simulink model "main_model"  (R2023b)
settings: Solver=FixedStepAuto  StartTime=0.0  StopTime=stopTime  RelTol=1e-3
values from neighbouring files (symbols this model uses):
  a = 6939    [Air_Drag_script.m]    (also in main.m = 6939.063; main_group24.m = 6978)
  A_BN0 = eye(3)    [main.m]
  c = 2.99792*10^8    (= 299792000)    [main.m]    (also in main_group24.m = 299792458)
  e = 0    [Air_Drag_script.m]    (also in main.m = 0.001304; main_group24.m)
  G = [gn, gm, gvali, gsvi]    [main.m]    (also in main_group24.m)
  H = [hn, hm, hvali, hsvi]    [main.m]    (also in main_group24.m)
  i = deg2rad(97.5307)    [Air_Drag_script.m]    (also in main.m; main_group24.m = deg2rad(98))
  inertia1 = Iz-Iy    (= -0.016811111)    [main.m]
  inertia2 = Ix-Iz    (= 0.033125546)    [main.m]
  inertia3 = Iy-Ix    (= -0.016314435)    [main.m]
  Inertia_matrix = [Ix 0 0; 0 Iy 0; 0 0 Iz]    [main.m]
  Inverse_inertia = inv(Inertia_matrix)    [main.m]
  m = [0.1; 0.1; 0.1]    [main.m]    (also in main_group24.m)
  MB = [4; 0.1; 0.1; 0.3]    [main.m]    (also in main_group24.m)
  mu = 3.98600433e+5    (= 398600.433)    [main.m]    (also in main_group24.m)
  n = 0.0011    [Air_Drag_script.m]    (also in main.m = sqrt(mu/a^3); main_group24.m = sqrt(mu/a^3))
  R_e = 6378    [main.m]    (also in main_group24.m)
  rho_d_MB = 0.1    [main.m]
  rho_d_SP = 0.1    [main.m]
  rho_s_MB = 0.5    [main.m]
  rho_s_SP = 0.1    [main.m]
  SP = [1; 0.3; 0.1; 0.01]    [main.m]    (also in main_group24.m = [0.25; 0.1; 0.3; 0.01])
  theta0 = deg2rad(30)    [main.m]    (also in main_group24.m = deg2rad(0))
  wx0 = deg2rad(3)    [main.m]    (also in main_group24.m)
  wy0 = deg2rad(11)    [main.m]    (also in main_group24.m)
  wz0 = deg2rad(14)    [main.m]    (also in main_group24.m)
libraries: matrix_library x8, vrlib x3, simulink_extras x1
(part 1 of 3)
settings Model: Creator=adity  LastModifiedBy=adity

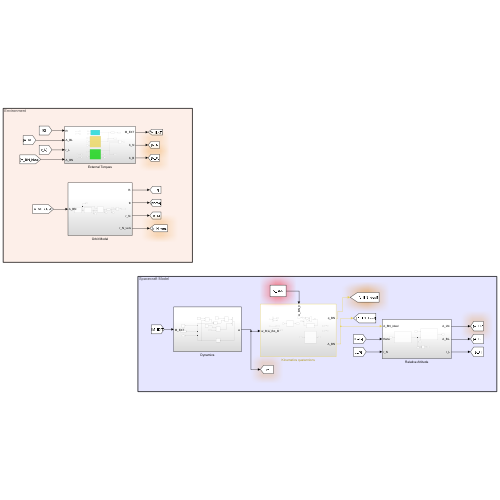
[thumbnail: Simulink's stored preview of the top-level diagram]
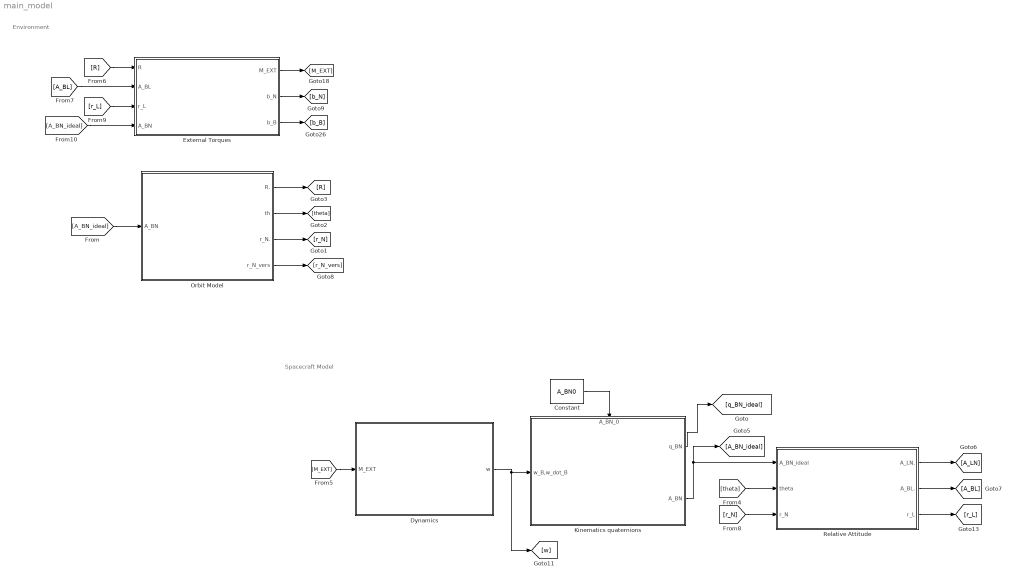
== system main_model ==
  note: Environment
  note: Spacecraft Model
  Constant : Constant  Value=A_BN0
  Dynamics : Subsystem
  External Torques : Subsystem
  Kinematics quaternions : Subsystem
      settings: PortSchema="{\"entries\":[{\"content\":{\"sides\":[{\"content\":{\"connectorIds\":[\"In1\"]},\"type\":\"ConnectorPlacement.EquallySpacedRectSide\",\"uuid\":\"b4580536-f47d-4a76-9d7a-ad9e45e6fd22\"},{\"content\":{\"connectorIds\":[\"Out1\",\"Out2\"],\"side\":\"RIGHT\"},\"type\":\"ConnectorPlacement.EquallySpacedRectSide\",\"uuid\":\"4273ed6e-d469-4a82-9e71-da4fb1c9f709\"},{\"content\":{\"connectorIds\":[\"In2\"],\"side\":\"TOP\"},\"type\":\"ConnectorPlacement.EquallySpacedRectSide\",\"uuid\":\"bac57a2b-a638-4d55-8f6f-550bb52319aa\"}]},\"type\":\"ConnectorPlacement.EquallySpacedConnector\",\"uuid\":\"29527554-7b77-4957-9d93-347c44cffae5\"}],\"packageUris\":[\"http://schema.mathworks.com/mf0/Connector/R2020b\"],\"version\":\"1.0\"}"
  Orbit Model : Subsystem
  Relative Attitude : Subsystem
  wires:
  [R] -> External Torques/1(R)
  [A_BL] -> External Torques/2(A_BL)
  [r_L] -> External Torques/3(r_L)
  [A_BN_ideal] -> Orbit Model/1(A_BN)
  [A_BN_ideal] -> External Torques/4(A_BN)
  External Torques/1(M_EXT) -> [M_EXT]
  Orbit Model/1(R.) -> [R]
  Orbit Model/3(r_N.) -> [r_N]
  Orbit Model/2(th) -> [theta]
  External Torques/2(b_N) -> [b_N]
  External Torques/3(b_B) -> [b_B]
  Orbit Model/4(r_N_vers) -> [r_N_vers]
  Relative Attitude/3(r_L) -> [r_L]
  [M_EXT] -> Dynamics/1(M_EXT)
  [r_N] -> Relative Attitude/3(r_N)
  Kinematics quaternions/2(A_BN) -> Relative Attitude/1(A_BN_ideal), [A_BN_ideal]
  [theta] -> Relative Attitude/2(theta)
  Dynamics/1(w) -> Kinematics quaternions/1(w_B,w_dot_B), [w]
  Relative Attitude/1(A_LN.) -> [A_LN]
  Relative Attitude/2(A_BL.) -> [A_BL]
  Kinematics quaternions/1(q_BN) -> [q_BN_ideal]
  Constant/1 -> Kinematics quaternions/2(A_BN_0)

== system main_model/Dynamics ==
  M_EXT : Inport
  Constant : Constant  Value=Inverse_inertia
  Constant1 : Constant  Value=Inertia_matrix
  Constant2 : Constant  Value=Inverse_inertia
  Cross Product : matrix_library/Cross Product
  Integrator : Integrator  InitialCondition=[wx0; wy0; wz0]
  MatrixMultiply : Product  Multiplication=Matrix(*)
  MatrixMultiply1 : Product  Multiplication=Matrix(*)
  MatrixMultiply2 : Product  Multiplication=Matrix(*)
  Scope : Scope
  Sum1 : Sum
  To Workspace : ToWorkspace  VariableName=w  SaveFormat=Timeseries  SampleTime=-1
  w : Outport
  wires:
  MatrixMultiply2/1 -> Sum1/2
  Sum1/1 -> Integrator/1
  Integrator/1 -> w/1, Scope/1, Cross Product/2, To Workspace/1, MatrixMultiply1/2
  Constant/1 -> MatrixMultiply/1
  Constant2/1 -> MatrixMultiply2/1
  MatrixMultiply/1 -> Sum1/1
  Constant1/1 -> MatrixMultiply1/1
  Cross Product/1 -> MatrixMultiply/2
  MatrixMultiply1/1 -> Cross Product/1
  M_EXT/1 -> MatrixMultiply2/2

== system main_model/External Torques ==
  R : Inport
  A_BL : Inport  Port=2
  r_L : Inport  Port=3
  A_BN : Inport  Port=4
  3D Norm2 : Subsystem
  Constant : Constant  Value=MB
  Constant1 : Constant  Value=SP
  M_GG : Subsystem
  Magnetic field : Subsystem
  Solar radiation : Subsystem
  Sum of Elements : Sum  Inputs=+++
  To Workspace : ToWorkspace  VariableName=M_GG  SaveFormat=Timeseries  SampleTime=-1
  To Workspace1 : ToWorkspace  VariableName=M_SRP  SaveFormat=Timeseries  SampleTime=-1
  To Workspace2 : ToWorkspace  VariableName=M_MAG  SaveFormat=Timeseries  SampleTime=-1
  M_EXT : Outport
  b_N : Outport  Port=2
  b_B : Outport  Port=3
  wires:
  [R] -> M_GG/2(R)
  Constant/1 -> Solar radiation/2(MB)
  Constant1/1 -> Solar radiation/3(SP)
  [A_BN] -> Solar radiation/1(A_BN)
  [A_BN] -> Magnetic field/2(A_BN)
  Magnetic field/1(M_MAG) -> To Workspace2/1, Sum of Elements/3
  Sum of Elements/1 -> M_EXT/1
  [A_BL] -> M_GG/1(A_BL)
  [r_L] -> Magnetic field/1(r_L)
  R/1 -> [R]
  A_BL/1 -> [A_BL]
  M_GG/1(M_GG1) -> Sum of Elements/1, 3D Norm2/1(V)
  r_L/1 -> [r_L]
  A_BN/1 -> [A_BN]
  Solar radiation/1(T_SRP) -> To Workspace1/1, Sum of Elements/2
  Magnetic field/2(b_N) -> b_N/1
  Magnetic field/3(b_B) -> b_B/1
  3D Norm2/1(normV) -> To Workspace/1

== system main_model/Kinematics quaternions ==
  w_B,w_dot_B : Inport
  A_BN_0 : Inport  Port=2
  DCM to quaternion : Subsystem
  Demux : Demux  Outputs=2
  Gain : Gain  Gain=1/2
  Integrator : Integrator  InitialConditionSource=external  InitialCondition=[0; 0; 0; 1]
  Matrix Multiply : Product  Multiplication=Matrix(*)
  Normalisation : Subsystem
  Reshape : Reshape  OutputDimensionality=Column vector (2-D)
  Subsystem : Subsystem
  Terminator : Terminator
  q to DCM : Subsystem
  q_BN : Outport
  A_BN : Outport  Port=2
  wires:
  [q_BN] -> q to DCM/1(q_BN)
  q to DCM/1(A_BN) -> [A_BN]
  [A_BN] -> A_BN/1
  [q_BN] -> q_BN/1
  [A_BN_0] -> DCM to quaternion/1(DCM)
  Matrix Multiply/1 -> Integrator/1  "dq/dt"
  Normalisation/1(Out1) -> [q_BN], Matrix Multiply/2  "q(t)"
  Gain/1 -> Matrix Multiply/1
  [OMEGA] -> Gain/1
  Integrator/1 -> Reshape/1  "q(t)"
  Reshape/1 -> Normalisation/1(In1)
  Subsystem/1(OMEGA) -> [OMEGA]
  DCM to quaternion/1(q) -> [q_0]
  [w_B] -> Subsystem/1(w_B)
  [q_0] -> Integrator/2
  A_BN_0/1 -> [A_BN_0]
  Demux/2 -> Terminator/1
  Demux/1 -> [w_B]
  w_B,w_dot_B/1 -> Demux/1

== system main_model/Orbit Model ==
  A_BN : Inport
  Normalize Vector : vrlib/Utilities/Normalize Vector  maxzero=0
  Product : Product  Multiplication=Matrix(*)
  R : Subsystem
  To Workspace1 : ToWorkspace  VariableName=r_B_vers  SampleTime=-1
  r_N : Subsystem
  theta : Subsystem
  R. : Outport
  th : Outport  Port=2
  r_N. : Outport  Port=3
  r_N_vers : Outport  Port=4
  wires:
  Normalize Vector/1 -> r_N_vers/1, Product/2
  r_N/1(r_N) -> r_N./1, Normalize Vector/1
  R/1(R) -> R./1, r_N/2(R)
  Product/1 -> To Workspace1/1
  theta/1(theta) -> th/1, r_N/1(theta), R/1(theta)
  A_BN/1 -> Product/1

== system main_model/Relative Attitude ==
  A_BN_ideal : Inport
  theta : Inport  Port=2
  r_N : Inport  Port=3
  A_BL : Subsystem
  A_LN : Subsystem
  MatrixMultiply : Product  Multiplication=Matrix(*)
  A_LN. : Outport
  A_BL. : Outport  Port=2
  r_L : Outport  Port=3
  wires:
  A_LN/1(A_LN) -> MatrixMultiply/1, A_LN./1, A_BL/2(A_LN)
  theta/1 -> A_LN/1(theta)
  A_BN_ideal/1 -> A_BL/1(A_BN)
  A_BL/1(A_BL) -> A_BL./1
  r_N/1 -> MatrixMultiply/2
  MatrixMultiply/1 -> r_L/1

== system main_model/External Torques/3D Norm2 ==
  V : Inport
  Add : Sum  Inputs=+++
  Demux : Demux  Outputs=3
  Square : Math  Operator=square
  Square Root : Sqrt
  Square1 : Math  Operator=square
  Square2 : Math  Operator=square
  normV : Outport
  wires:
  Square Root/1 -> normV/1
  V/1 -> Demux/1
  Demux/3 -> Square2/1
  Square/1 -> Add/1
  Demux/1 -> Square/1
  Demux/2 -> Square1/1
  Square2/1 -> Add/3
  Square1/1 -> Add/2
  Add/1 -> Square Root/1

== system main_model/External Torques/M_GG ==
  A_BL : Inport
  R : Inport  Port=2
  GG Torque1 : Subsystem
  "c1, c2, c3" : Subsystem
  M_GG1 : Outport
  wires:
  "c1, c2, c3"/1(c1) -> GG Torque1/1(c1)
  "c1, c2, c3"/2(c2) -> GG Torque1/2(c2)
  "c1, c2, c3"/3(c3) -> GG Torque1/3(c3)
  A_BL/1 -> "c1, c2, c3"/1(A_BL)
  GG Torque1/1(M_GG) -> M_GG1/1
  R/1 -> GG Torque1/4(R)

== system main_model/External Torques/Magnetic field ==
  r_L : Inport
  A_BN : Inport  Port=2
  Clock : Clock
  Constant : Constant  Value=m
  Constant1 : Constant  Value=R_e*1000
  Constant3 : Constant  Value=G
  Constant4 : Constant  Value=H
  Cross Product1 : matrix_library/Cross Product
  MATLAB Function : MATLAB Function  TreatAsAtomicUnit=on
  MatrixMultiply : Product  Multiplication=Matrix(*)
  Reshape1 : Reshape  OutputDimensionality=Column vector (2-D)
  M_MAG : Outport
  b_N : Outport  Port=2
  b_B : Outport  Port=3
  wires:
  Constant1/1 -> MATLAB Function/2(r)
  Clock/1 -> MATLAB Function/3(t)
  Constant3/1 -> MATLAB Function/4(G)
  MATLAB Function/1(b_N) -> Reshape1/1
  r_L/1 -> MATLAB Function/1(r_LVLH)
  Reshape1/1 -> b_N/1, MatrixMultiply/2
  Constant4/1 -> MATLAB Function/5(H)
  A_BN/1 -> MatrixMultiply/1
  Constant/1 -> Cross Product1/1
  MatrixMultiply/1 -> b_B/1, Cross Product1/2
  Cross Product1/1 -> M_MAG/1

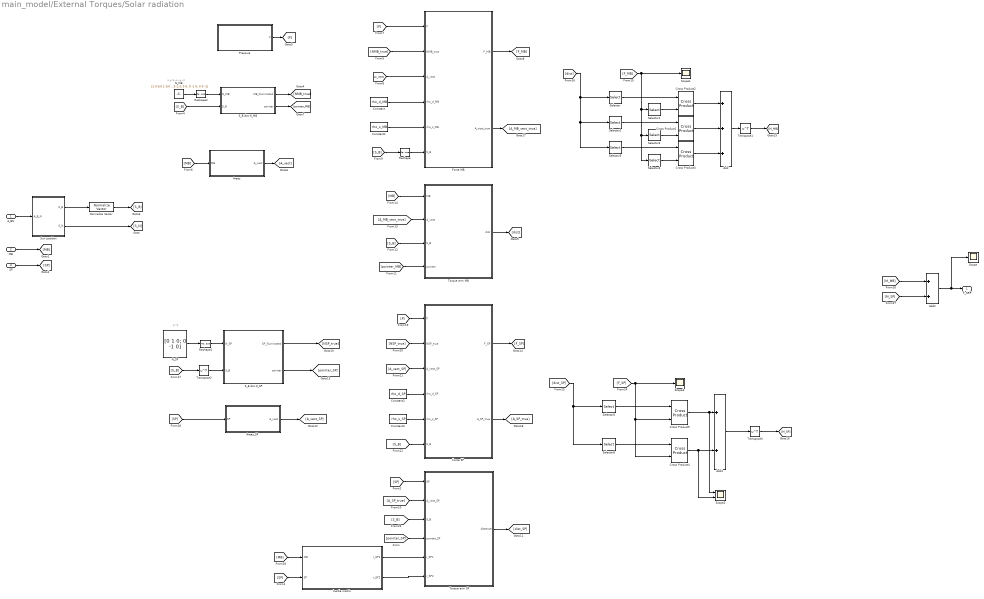
== system main_model/External Torques/Solar radiation ==
  note: x,y,z,-x,-y,-z
  note: y,-y
  A_BN : Inport
  MB : Inport  Port=2
  SP : Inport  Port=3
  Add : Sum  Inputs=3
  Add1 : Sum
  Add2 : Sum
  Areas : Subsystem
  Areas_SP : Subsystem
  Constant : Constant  Value=rho_d_MB
  Constant1 : Constant  Value=rho_s_MB
  Constant2 : Constant  Value=rho_d_SP
  Constant3 : Constant  Value=rho_s_SP
  Cross Product{1..5} (5 alike) : matrix_library/Cross Product
  Force MB : Subsystem
  Force SP : Subsystem
  Inertia matrix : Subsystem
  N_MB : Constant  Value=[1 0 0;0 1 0;0 0 1;-1 0 0; 0 -1 0; 0 0 -1]  VectorParams1D=off
  N_SP : Constant  Value=[0 1 0; 0 -1 0]  VectorParams1D=off
  Normalize Vector : vrlib/Utilities/Normalize Vector  maxzero=0
  Pressure : Subsystem
  Reshape : Reshape  OutputDimensionality=Column vector (2-D)
  Reshape1 : Reshape  OutputDimensionality=Customize  OutputDimensions=[2,3]
  Reshape2 : Reshape  OutputDimensionality=Customize  OutputDimensions=[6,3]
  S_B dot N_MB : Subsystem
  S_B dot N_SP : Subsystem
  Scope : Scope
  Scope1 : Scope
  Scope2 : Scope  NumInputPorts=2
  Scope3 : Scope
  Selector : Selector  NumberOfDimensions=2  InputPortWidth=3  IndexOptions=Index vector (dialog),Index vector (dialog)  Indices=1,[1 2 3]  OutputSizes=1,1
  Selector1 : Selector  NumberOfDimensions=2  InputPortWidth=3  IndexOptions=Index vector (dialog),Index vector (dialog)  Indices=1,[1 2 3]  OutputSizes=1,1
  Selector2 : Selector  NumberOfDimensions=2  InputPortWidth=3  IndexOptions=Index vector (dialog),Index vector (dialog)  Indices=2,[1 2 3]  OutputSizes=1,1
  Selector3 : Selector  NumberOfDimensions=2  InputPortWidth=3  IndexOptions=Index vector (dialog),Index vector (dialog)  Indices=2,[1 2 3]  OutputSizes=1,1
  Selector4 : Selector  NumberOfDimensions=2  InputPortWidth=3  IndexOptions=Index vector (dialog),Index vector (dialog)  Indices=3,[1 2 3]  OutputSizes=1,1
  Selector5 : Selector  NumberOfDimensions=2  InputPortWidth=3  IndexOptions=Index vector (dialog),Index vector (dialog)  Indices=3,[1 2 3]  OutputSizes=1,1
  Selector6 : Selector  NumberOfDimensions=2  InputPortWidth=3  IndexOptions=Index vector (dialog),Index vector (dialog)  Indices=1,[1 2 3]  OutputSizes=1,1
  Selector8 : Selector  NumberOfDimensions=2  InputPortWidth=3  IndexOptions=Index vector (dialog),Index vector (dialog)  Indices=2,[1 2 3]  OutputSizes=1,1
  Sun position : Subsystem
  Torque arm MB : Subsystem
  Torque arm SP : Subsystem
  Transpose1 : Math  Operator=transpose
  Transpose2 : Math  Operator=transpose
  Transpose3 : Math  Operator=transpose
  T_SRP : Outport
  wires:
  Sun position/1(S_B) -> Normalize Vector/1
  MB/1 -> [MB]
  N_MB/1 -> Reshape2/1
  [NMB_true] -> Force MB/2(NMB_true)
  S_B dot N_MB/1(MB_illuminated) -> [NMB_true]
  [MB] -> Areas/1(MB)
  [S_B] -> S_B dot N_MB/2(S_B)
  Sun position/2(S_N) -> [S_N]
  [P] -> Force MB/1(P)
  Areas/1(A_vect) -> [A_vect]
  Transpose1/1 -> [M_MB]
  Areas_SP/1(A_vect) -> [A_vect_SP]
  Reshape1/1 -> S_B dot N_SP/1(N_SP)
  Transpose3/1 -> [M_SP]
  Selector2/1 -> Cross Product1/1
  [MB] -> Torque arm MB/1(MB)
  Constant3/1 -> Force SP/5(rho_s_SP)
  [F_SP] -> Cross Product5/2, Cross Product4/2, Scope3/1
  [M_MB] -> Add2/1
  [dist_SP] -> Selector6/1, Selector8/1
  [pointer_SP] -> Torque arm SP/4(pointer_SP)
  Cross Product4/1 -> Scope2/2, Add1/2
  [F_MB] -> Scope1/1, Selector4/1, Selector3/1, Selector1/1
  A_BN/1 -> Sun position/1(A_B_N)
  Add1/1 -> Transpose3/1
  Transpose2/1 -> S_B dot N_SP/2(S_B)
  [SP] -> Areas_SP/1(SP)
  [A_SP_true] -> Torque arm SP/2(A_vect_SP)
  Add/1 -> Transpose1/1
  Torque arm SP/1(distance) -> [dist_SP]
  Reshape2/1 -> S_B dot N_MB/1(N_MB)
  Torque arm MB/1(dist) -> [dist]
  S_B dot N_SP/2(pointer) -> [pointer_SP]
  Force MB/1(F_MB) -> [F_MB]
  Selector/1 -> Cross Product2/1
  [S_B] -> Reshape/1
  [P] -> Force SP/1(P)
  [A_vect] -> Force MB/3(A_vect)
  Selector1/1 -> Cross Product2/2
  Constant1/1 -> Force MB/5(rho_s_MB)
  [A_MB_vect_true] -> Torque arm MB/2(A_vect)
  Pressure/1(P) -> [P]
  Normalize Vector/1 -> [S_B]
  Constant2/1 -> Force SP/4(rho_d_SP)
  Constant/1 -> Force MB/4(rho_d_MB)
  Selector8/1 -> Cross Product4/1
  [dist] -> Selector2/1, Selector5/1, Selector/1
  [NSP_true] -> Force SP/2(NSP_true)
  N_SP/1 -> Reshape1/1
  [S_B] -> Torque arm MB/3(S_B)
  Force SP/2(A_SP_true) -> [A_SP_true]
  [S_B] -> Torque arm SP/3(S_B)
  SP/1 -> [SP]
  Selector4/1 -> Cross Product3/2
  S_B dot N_MB/2(pointer) -> [pointer_MB]
  Force MB/2(A_vect_true) -> [A_MB_vect_true]
  [pointer_MB] -> Torque arm MB/4(pointer)
  Add2/1 -> Scope/1, T_SRP/1
  Selector3/1 -> Cross Product1/2
  [S_B] -> Force SP/6(S_B)
  [S_B] -> Transpose2/1
  Cross Product5/1 -> Scope2/1, Add1/1
  [A_vect_SP] -> Force SP/3(A_vect_SP)
  Reshape/1 -> Force MB/6(S_B)
  Cross Product2/1 -> Add/1
  Force SP/1(F_SP) -> [F_SP]
  S_B dot N_SP/1(SP_illuminated) -> [NSP_true]
  Selector6/1 -> Cross Product5/1
  Selector5/1 -> Cross Product3/1
  Cross Product1/1 -> Add/2
  [M_SP] -> Add2/2
  [SP] -> Torque arm SP/1(SP)
  Cross Product3/1 -> Add/3
  [SP] -> Inertia matrix/2(SP)
  [MB] -> Inertia matrix/1(MB)
  Inertia matrix/1(r_SP1) -> Torque arm SP/5(r_SP1)
  Inertia matrix/2(r_SP2) -> Torque arm SP/6(r_SP2)

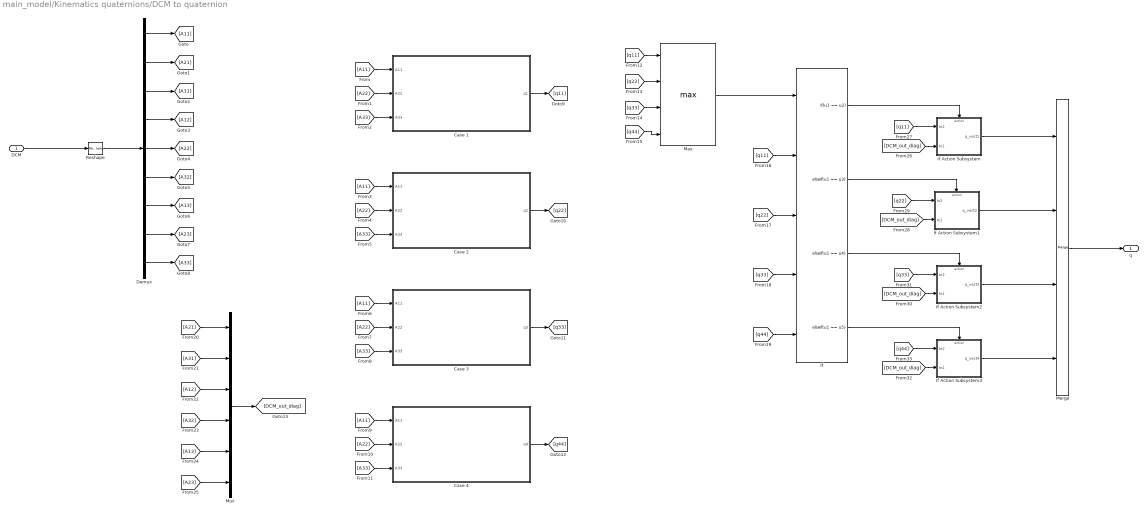
== system main_model/Kinematics quaternions/DCM to quaternion ==
  DCM : Inport
  Case 1 : Subsystem
  Case 2 : Subsystem
  Case 3 : Subsystem
  Case 4 : Subsystem
  Demux : Demux  Outputs=9
  If : If  NumInputs=5  IfExpression=u1 == u2  ElseIfExpressions=u1 == u3, u1 == u4, u1 == u5  ShowElse=off
  If Action Subsystem : Subsystem  TreatAsAtomicUnit=on
  If Action Subsystem1 : Subsystem  TreatAsAtomicUnit=on
  If Action Subsystem2 : Subsystem  TreatAsAtomicUnit=on
  If Action Subsystem3 : Subsystem  TreatAsAtomicUnit=on
  Max : MinMax  Function=max  Inputs=4
  Merge : Merge  Inputs=4
  Mux : Mux  Inputs=6
  Reshape : Reshape  OutputDimensionality=Column vector (2-D)
  q : Outport
  wires:
  [DCM_out_diag] -> If Action Subsystem3/2(In1)
  [q44] -> If Action Subsystem3/1(In2)
  [q33] -> If Action Subsystem2/1(In2)
  [DCM_out_diag] -> If Action Subsystem2/2(In1)
  [DCM_out_diag] -> If Action Subsystem1/2(In1)
  [q22] -> If Action Subsystem1/1(In2)
  [q11] -> If Action Subsystem/1(In2)
  [DCM_out_diag] -> If Action Subsystem/2(In1)
  Mux/1 -> [DCM_out_diag]
  [A21] -> Mux/1
  [A31] -> Mux/2
  [A12] -> Mux/3
  [A32] -> Mux/4
  [A13] -> Mux/5
  [A23] -> Mux/6
  Merge/1 -> q/1
  If Action Subsystem/1(q_vect1) -> Merge/1
  If Action Subsystem1/1(q_vect2) -> Merge/2
  If Action Subsystem2/1(q_vect3) -> Merge/3
  If Action Subsystem3/1(q_vect4) -> Merge/4
  If/4 -> If Action Subsystem3/Action
  If/3 -> If Action Subsystem2/Action
  If/2 -> If Action Subsystem1/Action
  If/1 -> If Action Subsystem/Action
  [q44] -> If/5
  [q33] -> If/4
  [q22] -> If/3
  [q11] -> If/2
  Max/1 -> If/1
  [q44] -> Max/4
  [q22] -> Max/2
  [q33] -> Max/3
  [q11] -> Max/1
  Case 4/1(q4) -> [q44]
  Case 3/1(q3) -> [q33]
  Case 2/1(q2) -> [q22]
  Case 1/1(q1) -> [q11]
  [A22] -> Case 4/2(A22)
  [A33] -> Case 4/3(A33)
  [A11] -> Case 4/1(A11)
  [A11] -> Case 3/1(A11)
  [A33] -> Case 3/3(A33)
  [A22] -> Case 3/2(A22)
  [A22] -> Case 2/2(A22)
  [A33] -> Case 2/3(A33)
  [A11] -> Case 2/1(A11)
  [A11] -> Case 1/1(A11)
  [A33] -> Case 1/3(A33)
  [A22] -> Case 1/2(A22)
  Demux/9 -> [A33]
  Demux/8 -> [A23]
  Demux/7 -> [A13]
  Demux/6 -> [A32]
  Demux/5 -> [A22]
  Demux/4 -> [A12]
  Demux/3 -> [A31]
  Demux/2 -> [A21]
  Demux/1 -> [A11]
  Reshape/1 -> Demux/1
  DCM/1 -> Reshape/1

== system main_model/Kinematics quaternions/Normalisation ==
  In1 : Inport
  Normalize Vector : vrlib/Utilities/Normalize Vector  maxzero=0
  Reshape : Reshape  OutputDimensionality=Column vector (2-D)
  Out1 : Outport
  wires:
  Reshape/1 -> Out1/1
  Normalize Vector/1 -> Reshape/1
  In1/1 -> Normalize Vector/1

== system main_model/Kinematics quaternions/Subsystem ==
  w_B : Inport
  Demux : Demux  Outputs=3
  Gain{1..6} (6 alike) : Gain  Gain=-1
  Ground : Ground
  Reshape : Reshape  OutputDimensionality=Customize  OutputDimensions=[4,4]
  Vector Concatenate : Concatenate  NumInputs=16
  OMEGA : Outport
  wires:
  [OMEGA] -> OMEGA/1
  Reshape/1 -> [OMEGA]
  [w_Bz] -> Vector Concatenate/15
  [w_By] -> Vector Concatenate/14
  [w_Bx] -> Vector Concatenate/13
  [w_Bz] -> Gain5/1
  [w_Bx] -> Vector Concatenate/10
  [w_By] -> Gain4/1
  [w_By] -> Gain3/1
  [w_Bx] -> Gain2/1
  [w_Bz] -> Vector Concatenate/5
  [w_Bx] -> Gain6/1
  [w_Bz] -> Gain1/1
  Gain1/1 -> Vector Concatenate/2
  Gain6/1 -> Vector Concatenate/4
  [w_By] -> Vector Concatenate/3
  Demux/3 -> [w_Bz]
  Demux/2 -> [w_By]
  Demux/1 -> [w_Bx]
  w_B/1 -> Demux/1
  Gain4/1 -> Vector Concatenate/9
  Vector Concatenate/1 -> Reshape/1
  Gain5/1 -> Vector Concatenate/12
  Gain2/1 -> Vector Concatenate/7
  Gain3/1 -> Vector Concatenate/8
  Ground/1 -> Vector Concatenate/16, Vector Concatenate/11, Vector Concatenate/6, Vector Concatenate/1

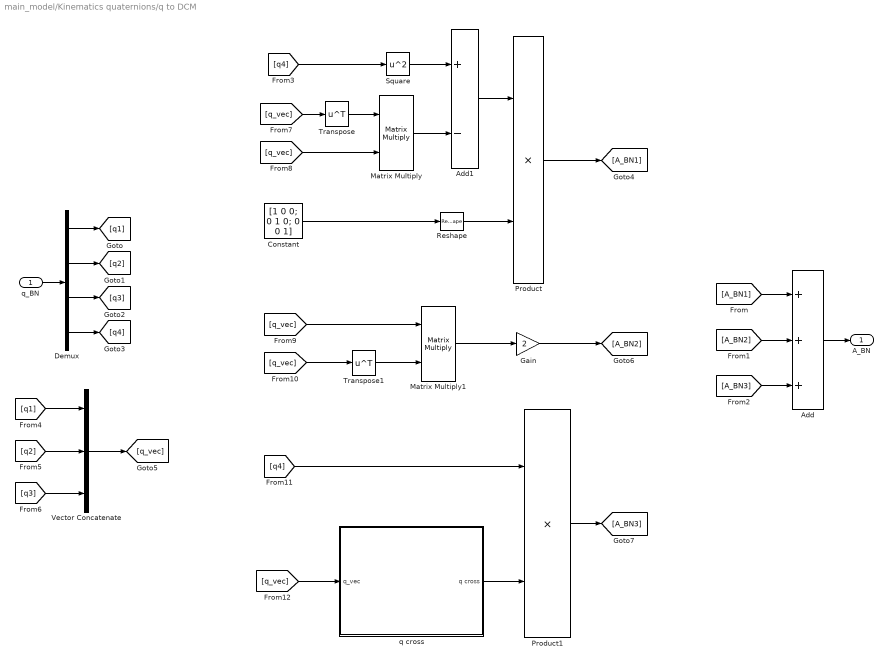
== system main_model/Kinematics quaternions/q to DCM ==
  q_BN : Inport
  Add : Sum  Inputs=+++
  Add1 : Sum  Inputs=+-
  Constant : Constant  Value=[1 0 0; 0 1 0; 0 0 1]
  Demux : Demux
  Gain : Gain  Gain=2
  Matrix Multiply : Product  Multiplication=Matrix(*)
  Matrix Multiply1 : Product  Multiplication=Matrix(*)
  Product : Product
  Product1 : Product
  Reshape : Reshape  OutputDimensionality=Customize  OutputDimensions=[3,3]
  Square : Math  Operator=square
  Transpose : Math  Operator=transpose
  Transpose1 : Math  Operator=transpose
  Vector Concatenate : Concatenate  NumInputs=3
  q cross : Subsystem
  A_BN : Outport
  wires:
  Product1/1 -> [A_BN3]
  q cross/1(q cross) -> Product1/2
  [q4] -> Product1/1
  [q_vec] -> q cross/1(q_vec)
  Gain/1 -> [A_BN2]
  Matrix Multiply1/1 -> Gain/1
  Transpose1/1 -> Matrix Multiply1/2
  [q_vec] -> Matrix Multiply1/1
  [q_vec] -> Transpose1/1
  Reshape/1 -> Product/2
  Constant/1 -> Reshape/1
  Add1/1 -> Product/1
  Product/1 -> [A_BN1]
  [q_vec] -> Matrix Multiply/2
  Transpose/1 -> Matrix Multiply/1
  Matrix Multiply/1 -> Add1/2
  [q_vec] -> Transpose/1
  Square/1 -> Add1/1
  [q4] -> Square/1
  Vector Concatenate/1 -> [q_vec]
  [q3] -> Vector Concatenate/3
  [q2] -> Vector Concatenate/2
  [q1] -> Vector Concatenate/1
  Add/1 -> A_BN/1
  [A_BN3] -> Add/3
  [A_BN2] -> Add/2
  [A_BN1] -> Add/1
  Demux/4 -> [q4]
  Demux/3 -> [q3]
  Demux/2 -> [q2]
  Demux/1 -> [q1]
  q_BN/1 -> Demux/1

== system main_model/Orbit Model/R ==
  theta : Inport
  Constant : Constant  Value=a
  Constant1 : Constant  Value=1-e^2
  Constant2 : Constant
  Constant3 : Constant  Value=e
  Cos : Trigonometry  Operator=cos
  Divide : Product  Inputs=*/
  Product : Product
  Product1 : Product
  Sum : Sum
  R : Outport
  wires:
  Sum/1 -> Divide/2
  Constant/1 -> Product/1
  Constant2/1 -> Sum/1
  Cos/1 -> Product1/2
  Product/1 -> Divide/1
  theta/1 -> Cos/1
  Divide/1 -> R/1
  Product1/1 -> Sum/2
  Constant3/1 -> Product1/1
  Constant1/1 -> Product/2

== system main_model/Orbit Model/r_N ==
  theta : Inport
  R : Inport  Port=2
  Constant : Constant  Value=cos(i)
  Constant1 : Constant  Value=sin(i)
  Cos : Trigonometry  Operator=cos
  Mux : Mux  Inputs=3
  Product : Product
  Product1 : Product
  Product2 : Product
  Sin : Trigonometry
  Sin1 : Trigonometry
  r_N : Outport
  wires:
  Constant/1 -> Product/2
  Cos/1 -> Mux/1
  Product/1 -> Mux/2
  Sin/1 -> Product/1
  Constant1/1 -> Product1/2
  Sin1/1 -> Product1/1
  Product1/1 -> Mux/3
  theta/1 -> Sin1/1, Cos/1, Sin/1
  Mux/1 -> Product2/2
  R/1 -> Product2/1
  Product2/1 -> r_N/1

== system main_model/Orbit Model/theta ==
  Constant : Constant
  Constant1 : Constant  Value=e
  Constant2 : Constant  Value=2
  Constant3 : Constant  Value=1-e^2
  Constant4 : Constant  Value=3/2
  Constant5 : Constant  Value=n
  Cos : Trigonometry  Operator=cos
  Divide : Product  Inputs=*/
  Integrator : Integrator  InitialCondition=theta0
  Pow : Math  Operator=pow  RndMeth=Zero
  Pow1 : Math  Operator=pow  RndMeth=Zero
  Product : Product
  Product1 : Product
  Sum : Sum
  To Workspace : ToWorkspace  VariableName=theta  SampleTime=-1
  theta : Outport
  wires:
  Cos/1 -> Product/2
  Constant/1 -> Sum/1
  Product/1 -> Sum/2
  Constant2/1 -> Pow/2
  Sum/1 -> Pow/1
  Constant1/1 -> Product/1
  Pow/1 -> Product1/2
  Product1/1 -> Divide/1
  Constant3/1 -> Pow1/1
  Constant4/1 -> Pow1/2
  Pow1/1 -> Divide/2
  Divide/1 -> Integrator/1
  Integrator/1 -> To Workspace/1, theta/1, Cos/1
  Constant5/1 -> Product1/1

== system main_model/Relative Attitude/A_BL ==
  A_BN : Inport
  A_LN : Inport  Port=2
  Matrix Multiply : Product  Multiplication=Matrix(*)
  To Workspace : ToWorkspace  VariableName=A_BL  SampleTime=-1
  Transpose1 : matrix_library/Transpose
  A_BL : Outport
  wires:
  A_BN/1 -> Matrix Multiply/1
  A_LN/1 -> Transpose1/1
  Transpose1/1 -> Matrix Multiply/2
  Matrix Multiply/1 -> A_BL/1, To Workspace/1

== system main_model/Relative Attitude/A_LN ==
  theta : Inport
  Constant : Constant  Value=0
  Constant1 : Constant  Value=[0; 0; 1]
  Constant2 : Constant  Value=[1 0 0; 0 cos(i) sin(i); 0 -sin(i) cos(i)]
  Cos : Trigonometry  Operator=cos
  Gain : Gain  Gain=[1; -1; 1]
  Matrix Concatenate : Concatenate  NumInputs=3  Mode=Multidimensional array  ConcatenateDimension=2
  Product : Product  Multiplication=Matrix(*)
  Selector : Selector  InputPortWidth=3  IndexOptions=Index vector (dialog)  Indices=[3 2 1]  OutputSizes=1
  Selector1 : Selector  InputPortWidth=3  IndexOptions=Index vector (dialog)  Indices=[2 3 1]  OutputSizes=1
  Sin : Trigonometry
  To Workspace : ToWorkspace  VariableName=A_LN  SampleTime=-1
  Vector Concatenate : Concatenate  NumInputs=3
  A_LN : Outport
  wires:
  Matrix Concatenate/1 -> Product/1
  theta/1 -> Sin/1, Cos/1
  Gain/1 -> Matrix Concatenate/1
  Vector Concatenate/1 -> Selector1/1, Selector/1
  Sin/1 -> Vector Concatenate/3
  Selector/1 -> Matrix Concatenate/2
  Selector1/1 -> Gain/1
  Product/1 -> A_LN/1, To Workspace/1
  Constant1/1 -> Matrix Concatenate/3
  Cos/1 -> Vector Concatenate/2
  Constant/1 -> Vector Concatenate/1
  Constant2/1 -> Product/2

== system main_model/External Torques/M_GG/GG Torque1 ==
  c1 : Inport
  c2 : Inport  Port=2
  c3 : Inport  Port=3
  R : Inport  Port=4
  Constant : Constant  Value=3
  Divide : Product  Inputs=*/
  Divide1 : Product  Inputs=*/
  Divide2 : Product  Inputs=*/
  Gain4 : Gain  Gain=3*mu
  Gain5 : Gain  Gain=3*mu
  Gain7 : Gain  Gain=3*mu
  Ix-Iz : Gain  Gain=inertia2
  Iy-Ix : Gain  Gain=inertia3
  Iz-Iy : Gain  Gain=inertia1
  Mux : Mux  Inputs=3
  Pow : Math  Operator=pow  RndMeth=Zero
  Product3 : Product
  Product4 : Product
  Product5 : Product
  M_GG : Outport
  wires:
  Pow/1 -> Divide2/2, Divide1/2, Divide/2
  Iz-Iy/1 -> Mux/1
  c3/1 -> Product3/2, Product4/2
  Product3/1 -> Gain4/1
  Divide2/1 -> Iy-Ix/1
  Gain4/1 -> Divide/1
  Gain5/1 -> Divide1/1
  Divide/1 -> Iz-Iy/1
  Constant/1 -> Pow/2
  Divide1/1 -> Ix-Iz/1
  Product5/1 -> Gain7/1
  c1/1 -> Product5/1, Product4/1
  R/1 -> Pow/1
  Iy-Ix/1 -> Mux/3
  Ix-Iz/1 -> Mux/2
  Gain7/1 -> Divide2/1
  Product4/1 -> Gain5/1
  c2/1 -> Product3/1, Product5/2
  Mux/1 -> M_GG/1

== system main_model/External Torques/M_GG/c1, c2, c3 ==
  A_BL : Inport
  Constant1 : Constant  Value=[1; 0; 0]
  Demux : Demux  Outputs=3
  Product1 : Product  Multiplication=Matrix(*)
  c1 : Outport
  c2 : Outport  Port=2
  c3 : Outport  Port=3
  wires:
  Demux/2 -> c2/1
  Product1/1 -> Demux/1
  Demux/1 -> c1/1
  Demux/3 -> c3/1
  Constant1/1 -> Product1/2
  A_BL/1 -> Product1/1

== system main_model/External Torques/Solar radiation/Areas ==
  MB : Inport
  Demux : Demux
  Mux : Mux  Inputs=3
  Product1 : Product
  Product2 : Product
  Product4 : Product
  Reshape : Reshape  OutputDimensionality=Column vector (2-D)
  Terminator : Terminator
  A_vect : Outport
  wires:
  Product2/1 -> Mux/2  "a*h"
  Product4/1 -> Mux/1  "b*h"
  MB/1 -> Demux/1
  Product1/1 -> Mux/3  "a*b"
  Demux/1 -> Terminator/1
  Demux/2 -> [a]
  Demux/3 -> [b]
  Demux/4 -> [h]
  [b] -> Product4/1
  [h] -> Product4/2
  [h] -> Product2/2
  [b] -> Product1/2
  [a] -> Product2/1
  [a] -> Product1/1
  Mux/1 -> Reshape/1
  Reshape/1 -> A_vect/1

== system main_model/External Torques/Solar radiation/Areas_SP ==
  SP : Inport
  Demux : Demux
  Product1 : Product
  Terminator : Terminator
  Terminator1 : Terminator
  A_vect : Outport
  wires:
  [a] -> Product1/1
  [b] -> Product1/2
  Demux/4 -> Terminator1/1
  Demux/3 -> [b]
  Demux/2 -> [a]
  Demux/1 -> Terminator/1
  Product1/1 -> A_vect/1  "a*b"
  SP/1 -> Demux/1

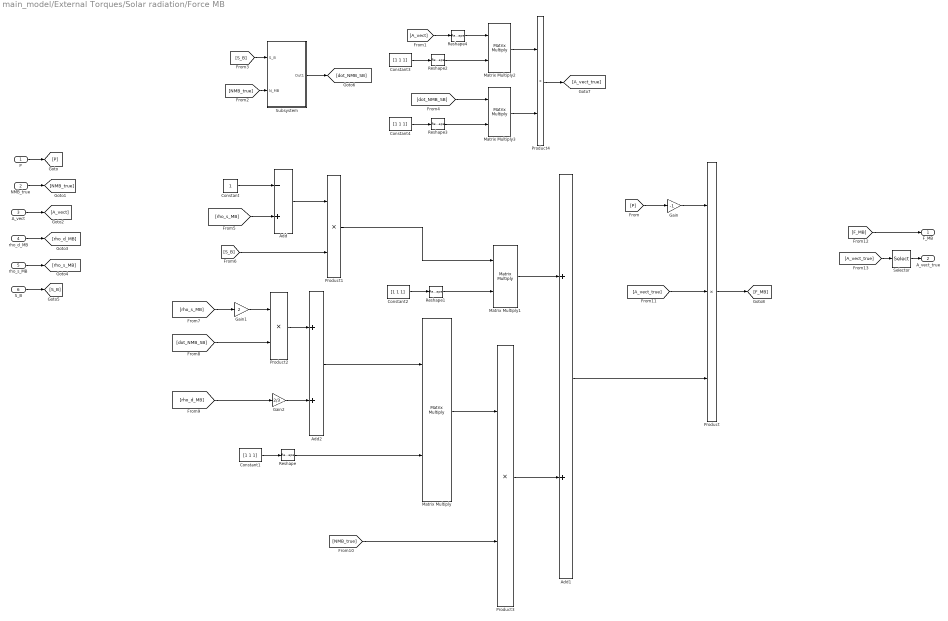
== system main_model/External Torques/Solar radiation/Force MB ==
  P : Inport
  NMB_true : Inport  Port=2
  A_vect : Inport  Port=3
  rho_d_MB : Inport  Port=4
  rho_s_MB : Inport  Port=5
  S_B : Inport  Port=6
  Add : Sum  Inputs=-+
  Add1 : Sum
  Add2 : Sum
  Constant : Constant
  Constant{1..4} (4 alike) : Constant  Value=[1 1 1]
  Gain : Gain  Gain=-1
  Gain1 : Gain  Gain=2
  Gain2 : Gain  Gain=2/3
  Matrix Multiply{,1..3} (4 alike) : Product  Multiplication=Matrix(*)
  Product : Product  Inputs=3
  Product{1..4} (4 alike) : Product
  Reshape{,1..3} (4 alike) : Reshape  OutputDimensionality=Row vector (2-D)
  Reshape4 : Reshape  OutputDimensionality=Column vector (2-D)
  Selector : Selector  NumberOfDimensions=2  InputPortWidth=3  IndexOptions=Index vector (dialog),Index vector (dialog)  Indices=[1 2 3],1  OutputSizes=1,1
  Subsystem : Subsystem
  F_MB : Outport
  A_vect_true : Outport  Port=2
  wires:
  P/1 -> [P]
  NMB_true/1 -> [NMB_true]
  A_vect/1 -> [A_vect]
  rho_d_MB/1 -> [rho_d_MB]
  rho_s_MB/1 -> [rho_s_MB]
  S_B/1 -> [S_B]
  [P] -> Gain/1
  Gain/1 -> Product/1
  [NMB_true] -> Subsystem/2(N_MB)
  [S_B] -> Subsystem/1(S_B)
  Subsystem/1(Out1) -> [dot_NMB_SB]
  [rho_s_MB] -> Add/2
  Constant/1 -> Add/1
  Add/1 -> Product1/1
  [S_B] -> Product1/2
  [rho_s_MB] -> Gain1/1
  [dot_NMB_SB] -> Product2/2
  Gain1/1 -> Product2/1
  Product2/1 -> Add2/1
  Gain2/1 -> Add2/2
  [rho_d_MB] -> Gain2/1
  [NMB_true] -> Product3/2
  Product3/1 -> Add1/2
  Add1/1 -> Product/3
  Constant1/1 -> Reshape/1
  Matrix Multiply/1 -> Product3/1
  Add2/1 -> Matrix Multiply/1
  Reshape/1 -> Matrix Multiply/2
  Matrix Multiply1/1 -> Add1/1
  Product1/1 -> Matrix Multiply1/1
  Constant2/1 -> Reshape1/1
  Reshape1/1 -> Matrix Multiply1/2
  Reshape2/1 -> Matrix Multiply2/2
  Constant3/1 -> Reshape2/1
  Reshape3/1 -> Matrix Multiply3/2
  Constant4/1 -> Reshape3/1
  [A_vect] -> Reshape4/1
  Reshape4/1 -> Matrix Multiply2/1
  [dot_NMB_SB] -> Matrix Multiply3/1
  Matrix Multiply2/1 -> Product4/1
  Matrix Multiply3/1 -> Product4/2
  Product4/1 -> [A_vect_true]
  [A_vect_true] -> Product/2
  Product/1 -> [F_MB]
  [F_MB] -> F_MB/1
  [A_vect_true] -> Selector/1
  Selector/1 -> A_vect_true/1

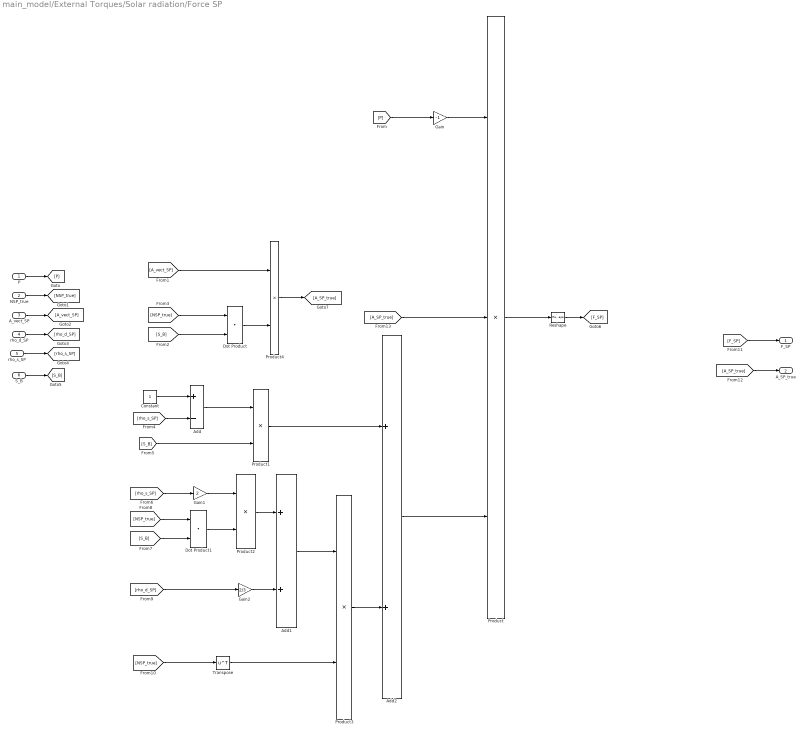
== system main_model/External Torques/Solar radiation/Force SP ==
  P : Inport
  NSP_true : Inport  Port=2
  A_vect_SP : Inport  Port=3
  rho_d_SP : Inport  Port=4
  rho_s_SP : Inport  Port=5
  S_B : Inport  Port=6
  Add : Sum  Inputs=+-
  Add1 : Sum
  Add2 : Sum
  Constant : Constant
  Dot Product : DotProduct  OutDataTypeStr=Inherit: Inherit via internal rule
  Dot Product1 : DotProduct  OutDataTypeStr=Inherit: Inherit via internal rule
  Gain : Gain  Gain=-1
  Gain1 : Gain  Gain=2
  Gain2 : Gain  Gain=2/3
  Product : Product  Inputs=3
  Product{1..4} (4 alike) : Product
  Reshape : Reshape  OutputDimensionality=Row vector (2-D)
  Transpose : Math  Operator=transpose
  F_SP : Outport
  A_SP_true : Outport  Port=2
  wires:
  P/1 -> [P]
  NSP_true/1 -> [NSP_true]
  A_vect_SP/1 -> [A_vect_SP]
  rho_d_SP/1 -> [rho_d_SP]
  rho_s_SP/1 -> [rho_s_SP]
  S_B/1 -> [S_B]
  Product/1 -> Reshape/1
  [P] -> Gain/1
  Gain/1 -> Product/1
  [S_B] -> Dot Product/2
  [NSP_true] -> Dot Product/1
  Constant/1 -> Add/1
  [rho_s_SP] -> Add/2
  Add/1 -> Product1/1
  [S_B] -> Product1/2
  [rho_s_SP] -> Gain1/1
  [NSP_true] -> Dot Product1/1
  [S_B] -> Dot Product1/2
  Dot Product1/1 -> Product2/2
  Gain1/1 -> Product2/1
  Product2/1 -> Add1/1
  [rho_d_SP] -> Gain2/1
  Gain2/1 -> Add1/2
  [NSP_true] -> Transpose/1
  Add1/1 -> Product3/1
  Product1/1 -> Add2/1
  Product3/1 -> Add2/2
  Transpose/1 -> Product3/2
  Add2/1 -> Product/3
  Reshape/1 -> [F_SP]
  [F_SP] -> F_SP/1
  Dot Product/1 -> Product4/2
  [A_vect_SP] -> Product4/1
  Product4/1 -> [A_SP_true]
  [A_SP_true] -> A_SP_true/1
  [A_SP_true] -> Product/2

== system main_model/External Torques/Solar radiation/Inertia matrix ==
  MB : Inport
  SP : Inport  Port=2
  Demux : Demux
  Demux1 : Demux
  Terminator{,1..5} (6 alike) : Terminator
  r_SP : Subsystem
  r_SP1 : Outport
  r_SP2 : Outport  Port=2
  wires:
  [a_MB] -> r_SP/2(a_MB)
  Demux/1 -> Terminator5/1
  SP/1 -> Demux/1
  Demux1/2 -> [a_MB]
  Demux1/3 -> Terminator/1
  Demux1/1 -> Terminator2/1
  Demux1/4 -> Terminator1/1
  MB/1 -> Demux1/1
  Demux/4 -> Terminator3/1
  Demux/2 -> Terminator4/1
  r_SP/2(r_SP2) -> r_SP2/1
  Demux/3 -> [b_SP]
  [b_SP] -> r_SP/1(b_SP)
  r_SP/1(r_SP1) -> r_SP1/1

== system main_model/External Torques/Solar radiation/Pressure ==
  Constant6 : Constant  Value=1358
  Constant7 : Constant  Value=c
  Product8 : Product
  Reciprocal : Product  Inputs=/
  P : Outport
  wires:
  Constant6/1 -> Product8/1
  Reciprocal/1 -> Product8/2
  Product8/1 -> P/1
  Constant7/1 -> Reciprocal/1

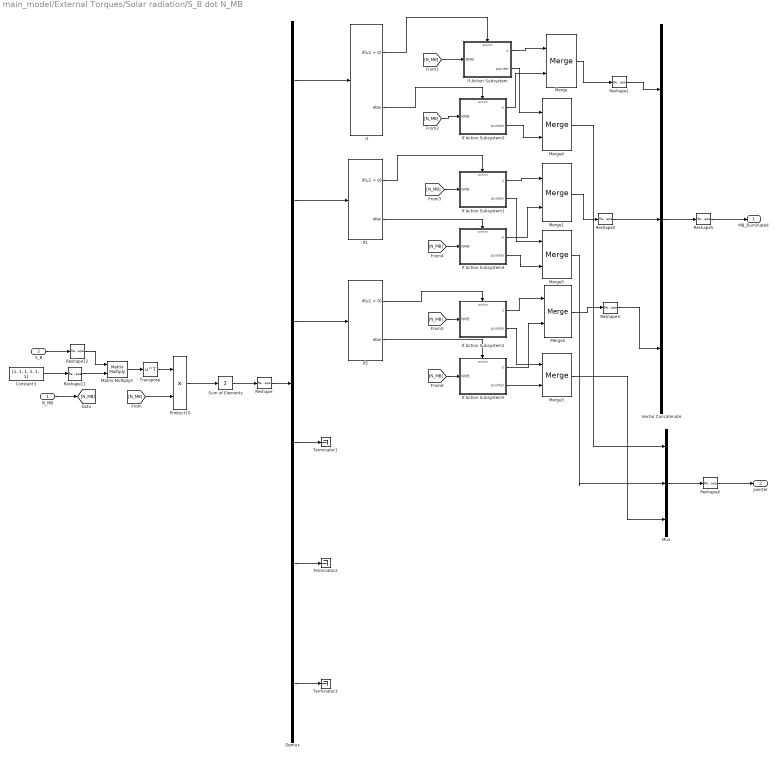
== system main_model/External Torques/Solar radiation/S_B dot N_MB ==
  N_MB : Inport
  S_B : Inport  Port=2
  Constant3 : Constant  Value=[1, 1, 1, 1, 1, 1]  VectorParams1D=off
  Demux : Demux  Outputs=6
  If : If
  If Action Subsystem : Subsystem  TreatAsAtomicUnit=on
  If Action Subsystem1 : Subsystem  TreatAsAtomicUnit=on
  If Action Subsystem2 : Subsystem  TreatAsAtomicUnit=on
  If Action Subsystem3 : Subsystem  TreatAsAtomicUnit=on
  If Action Subsystem4 : Subsystem  TreatAsAtomicUnit=on
  If Action Subsystem5 : Subsystem  TreatAsAtomicUnit=on
  If1 : If
  If2 : If
  Matrix Multiply5 : Product  Multiplication=Matrix(*)
  Merge{,1..5} (6 alike) : Merge
  Mux : Mux  Inputs=3
  Product10 : Product
  Reshape{,1..4,12} (6 alike) : Reshape  OutputDimensionality=Column vector (2-D)
  Reshape11 : Reshape  OutputDimensionality=Row vector (2-D)
  Reshape5 : Reshape  OutputDimensionality=Customize  OutputDimensions=[3,3]
  Sum of Elements : Sum  Inputs=+  CollapseMode=Specified dimension  CollapseDim=2
  Terminator1 : Terminator
  Terminator2 : Terminator
  Terminator3 : Terminator
  Transpose : Math  Operator=transpose
  Vector Concatenate : Concatenate  NumInputs=3
  MB_illuminated : Outport
  pointer : Outport  Port=2
  wires:
  Reshape12/1 -> Matrix Multiply5/1
  Matrix Multiply5/1 -> Transpose/1
  Product10/1 -> Sum of Elements/1
  Reshape11/1 -> Matrix Multiply5/2
  Constant3/1 -> Reshape11/1
  S_B/1 -> Reshape12/1
  Sum of Elements/1 -> Reshape/1
  Reshape/1 -> Demux/1
  Demux/1 -> If/1
  If/1 -> If Action Subsystem/Action
  If/2 -> If Action Subsystem3/Action
  N_MB/1 -> [N_MB]
  [N_MB] -> Product10/2
  [N_MB] -> If Action Subsystem/1(NMB)
  Demux/4 -> Terminator1/1
  Demux/5 -> Terminator2/1
  Demux/6 -> Terminator3/1
  Demux/2 -> If1/1
  If1/1 -> If Action Subsystem1/Action
  [N_MB] -> If Action Subsystem3/1(NMB)
  [N_MB] -> If Action Subsystem1/1(NMB)
  If1/2 -> If Action Subsystem4/Action
  [N_MB] -> If Action Subsystem4/1(NMB)
  If Action Subsystem3/1(-x) -> Merge/2
  If Action Subsystem/1(x) -> Merge/1
  If Action Subsystem1/1(y) -> Merge1/1
  If Action Subsystem2/1(z) -> Merge2/1
  If Action Subsystem5/1(-z) -> Merge2/2
  Demux/3 -> If2/1
  If2/1 -> If Action Subsystem2/Action
  If2/2 -> If Action Subsystem5/Action
  [N_MB] -> If Action Subsystem2/1(NMB)
  [N_MB] -> If Action Subsystem5/1(NMB)
  Merge/1 -> Reshape1/1
  Merge1/1 -> Reshape2/1
  Merge2/1 -> Reshape3/1
  Reshape1/1 -> Vector Concatenate/1
  Reshape2/1 -> Vector Concatenate/2
  Reshape3/1 -> Vector Concatenate/3
  Vector Concatenate/1 -> Reshape5/1
  If Action Subsystem4/1(-y) -> Merge1/2
  If Action Subsystem/2(pointer) -> Merge4/1
  If Action Subsystem3/2(pointer) -> Merge4/2
  If Action Subsystem1/2(pointer) -> Merge5/1
  If Action Subsystem4/2(pointer) -> Merge5/2
  If Action Subsystem2/2(pointer) -> Merge3/1
  If Action Subsystem5/2(pointer) -> Merge3/2
  Merge4/1 -> Mux/1
  Merge5/1 -> Mux/2
  Merge3/1 -> Mux/3
  Mux/1 -> Reshape4/1
  Reshape4/1 -> pointer/1
  Reshape5/1 -> MB_illuminated/1
  Transpose/1 -> Product10/1

== system main_model/External Torques/Solar radiation/S_B dot N_SP ==
  N_SP : Inport
  S_B : Inport  Port=2
  Constant3 : Constant  Value=[1, 1]
  Demux : Demux  Outputs=2
  If : If
  If Action Subsystem : Subsystem  TreatAsAtomicUnit=on
  If Action Subsystem1 : Subsystem  TreatAsAtomicUnit=on
  If1 : If
  Matrix Multiply5 : Product  Multiplication=Matrix(*)
  Merge : Merge
  Merge1 : Merge
  Product10 : Product
  Reshape11 : Reshape  OutputDimensionality=Row vector (2-D)
  Reshape12 : Reshape  OutputDimensionality=Column vector (2-D)
  Sum of Elements : Sum  Inputs=+  CollapseMode=Specified dimension  CollapseDim=2
  Terminator : Terminator
  Terminator1 : Terminator
  Transpose : Math  Operator=transpose
  SP_illuminated : Outport
  pointer : Outport  Port=2
  wires:
  [N_SP] -> Product10/2
  N_SP/1 -> [N_SP]
  Sum of Elements/1 -> Demux/1
  S_B/1 -> Reshape12/1
  Constant3/1 -> Reshape11/1
  Reshape11/1 -> Matrix Multiply5/2
  Product10/1 -> Sum of Elements/1
  Matrix Multiply5/1 -> Transpose/1
  Reshape12/1 -> Matrix Multiply5/1
  Transpose/1 -> Product10/1
  Demux/1 -> If/1
  If/1 -> If Action Subsystem/Action
  Demux/2 -> If1/1
  [N_SP] -> If Action Subsystem/1(N_SP)
  [N_SP] -> If Action Subsystem1/1(N_SP)
  If1/1 -> If Action Subsystem1/Action
  If1/2 -> Terminator/1
  If/2 -> Terminator1/1
  If Action Subsystem/1(true_NSP) -> Merge/1
  If Action Subsystem1/1(true_NSP) -> Merge/2
  If Action Subsystem/2(pointer) -> Merge1/1
  If Action Subsystem1/2(pointer) -> Merge1/2
  Merge/1 -> SP_illuminated/1
  Merge1/1 -> pointer/1

== system main_model/External Torques/Solar radiation/Sun position ==
  A_B_N : Inport
  Clock : Clock
  Constant : Constant  Value=2*pi
  Constant1 : Constant  Value=365*24*60*60
  Constant2 : Constant  Value=23.45
  Degrees to Radians : simulink_extras/Transformations/Degrees to Radians
  MatrixMultiply : Product  Multiplication=Matrix(*)
  Mux : Mux  Inputs=3
  Product{,1..3} (4 alike) : Product
  Reciprocal : Product  Inputs=1
  Reshape : Reshape  OutputDimensionality=Column vector (2-D)
  Sin : Trigonometry  Operator=cos
  Sin1 : Trigonometry
  Sin2 : Trigonometry  Operator=cos
  Sin3 : Trigonometry
  S_B : Outport
  S_N : Outport  Port=2
  wires:
  Product3/1 -> Mux/3
  Degrees to Radians/1 -> Sin3/1, Sin2/1
  Constant1/1 -> Reciprocal/1
  Sin2/1 -> Product2/2
  Product/1 -> Product1/1  "n"
  Constant2/1 -> Degrees to Radians/1
  Product1/1 -> Sin/1, Sin1/1  "n*t"
  Product2/1 -> Mux/2
  Sin3/1 -> Product3/2
  Clock/1 -> Product1/2
  Sin1/1 -> Product3/1, Product2/1
  Constant/1 -> Product/1
  Sin/1 -> Mux/1
  Reciprocal/1 -> Product/2
  Mux/1 -> Reshape/1
  A_B_N/1 -> MatrixMultiply/1
  MatrixMultiply/1 -> S_B/1
  Reshape/1 -> S_N/1, MatrixMultiply/2

== system main_model/External Torques/Solar radiation/Torque arm MB ==
  note: creo il vettore somma che ha per colonna i raggi vettori che collegano il CM del MB con i centri illuminati delle facce nel caso che il sole sia nelle 4 posizioni.
  MB : Inport
  A_vect : Inport  Port=2
  S_B : Inport  Port=3
  pointer : Inport  Port=4
  Demux : Demux  Outputs=3
  Reshape : Reshape  OutputDimensionality=Customize  OutputDimensions=[3,3]
  Transpose : Math  Operator=transpose
  Vector Concatenate : Concatenate  NumInputs=3
  creazione raggi vettore tra CM MB e centro facce illuminate della faccia che ha come normale l'asse i : Subsystem
  creazione raggi vettore tra CM MB e centro facce illuminate della faccia che ha come normale l'asse j : Subsystem
  creazione raggi vettore tra CM MB e centro facce illuminate della faccia che ha come normale l'asse k : Subsystem
  dist : Outport
  wires:
  pointer/1 -> Demux/1
  [x] -> creazione raggi vettore tra CM MB e centro facce illuminate della faccia che ha come normale l'asse i/4(pointer)
  [A_vect] -> creazione raggi vettore tra CM MB e centro facce illuminate della faccia che ha come normale l'asse i/3(A_vect)
  [MB] -> creazione raggi vettore tra CM MB e centro facce illuminate della faccia che ha come normale l'asse k/2(MB)
  [y] -> creazione raggi vettore tra CM MB e centro facce illuminate della faccia che ha come normale l'asse j/4(pointer)
  S_B/1 -> [S_B]
  [A_vect] -> creazione raggi vettore tra CM MB e centro facce illuminate della faccia che ha come normale l'asse k/3(A_vect)
  [MB] -> creazione raggi vettore tra CM MB e centro facce illuminate della faccia che ha come normale l'asse j/2(MB)
  A_vect/1 -> [A_vect]
  MB/1 -> [MB]
  [MB] -> creazione raggi vettore tra CM MB e centro facce illuminate della faccia che ha come normale l'asse i/2(MB)
  Reshape/1 -> Transpose/1
  Transpose/1 -> dist/1
  [S_B] -> creazione raggi vettore tra CM MB e centro facce illuminate della faccia che ha come normale l'asse k/1(S_B)
  Demux/1 -> [x]
  Demux/3 -> [z]
  [S_B] -> creazione raggi vettore tra CM MB e centro facce illuminate della faccia che ha come normale l'asse j/1(S_B)
  [z] -> creazione raggi vettore tra CM MB e centro facce illuminate della faccia che ha come normale l'asse k/4(pointer)
  Vector Concatenate/1 -> Reshape/1  "vectors x, y, z"
  [A_vect] -> creazione raggi vettore tra CM MB e centro facce illuminate della faccia che ha come normale l'asse j/3(A_vect)
  [S_B] -> creazione raggi vettore tra CM MB e centro facce illuminate della faccia che ha come normale l'asse i/1(S_B)
  Demux/2 -> [y]
  creazione raggi vettore tra CM MB e centro facce illuminate della faccia che ha come normale l'asse k/1(Out1) -> Vector Concatenate/3
  creazione raggi vettore tra CM MB e centro facce illuminate della faccia che ha come normale l'asse j/1(Out1) -> Vector Concatenate/2
  creazione raggi vettore tra CM MB e centro facce illuminate della faccia che ha come normale l'asse i/1(Out1) -> Vector Concatenate/1

== system main_model/External Torques/Solar radiation/Torque arm SP ==
  SP : Inport
  A_vect_SP : Inport  Port=2
  S_B : Inport  Port=3
  pointer_SP : Inport  Port=4
  r_SP1 : Inport  Port=5
  r_SP2 : Inport  Port=6
  Add : Sum
  Add1 : Sum
  Reshape : Reshape  OutputDimensionality=Customize  OutputDimensions=[2,3]
  Vector Concatenate : Concatenate
  creazione raggi vettore tra CM SP e centro facce illuminate della faccia che ha come normale l'asse j : Subsystem
  distance : Outport
  wires:
  Reshape/1 -> distance/1
  SP/1 -> [SP]
  A_vect_SP/1 -> [A_vect_SP]
  S_B/1 -> [S_B]
  pointer_SP/1 -> [pointer_SP]
  r_SP1/1 -> [r_SP1]
  r_SP2/1 -> [r_SP2]
  [S_B] -> creazione raggi vettore tra CM SP e centro facce illuminate della faccia che ha come normale l'asse j/1(S_B)
  [SP] -> creazione raggi vettore tra CM SP e centro facce illuminate della faccia che ha come normale l'asse j/2(SP)
  [A_vect_SP] -> creazione raggi vettore tra CM SP e centro facce illuminate della faccia che ha come normale l'asse j/3(A_vect)
  [pointer_SP] -> creazione raggi vettore tra CM SP e centro facce illuminate della faccia che ha come normale l'asse j/4(pointer)
  creazione raggi vettore tra CM SP e centro facce illuminate della faccia che ha come normale l'asse j/1(distance) -> [distance]
  Vector Concatenate/1 -> Reshape/1
  Add/1 -> Vector Concatenate/1
  [distance] -> Add/1
  [r_SP1] -> Add/2
  [r_SP2] -> Add1/2
  [distance] -> Add1/1
  Add1/1 -> Vector Concatenate/2

== system main_model/Kinematics quaternions/DCM to quaternion/Case 1 ==
  A11 : Inport
  A22 : Inport  Port=2
  A33 : Inport  Port=3
  Add : Sum  Inputs=++--
  Constant : Constant
  Gain : Gain  Gain=1/2
  Sqrt : Sqrt
  q1 : Outport
  wires:
  Gain/1 -> q1/1
  Sqrt/1 -> Gain/1
  Add/1 -> Sqrt/1
  Constant/1 -> Add/1
  A33/1 -> Add/4
  A11/1 -> Add/2
  A22/1 -> Add/3

== system main_model/Kinematics quaternions/DCM to quaternion/Case 2 ==
  A11 : Inport
  A22 : Inport  Port=2
  A33 : Inport  Port=3
  Add : Sum  Inputs=+-+-
  Constant : Constant
  Gain : Gain  Gain=1/2
  Sqrt : Sqrt
  q2 : Outport
  wires:
  A22/1 -> Add/3
  A11/1 -> Add/2
  A33/1 -> Add/4
  Constant/1 -> Add/1
  Add/1 -> Sqrt/1
  Sqrt/1 -> Gain/1
  Gain/1 -> q2/1

== system main_model/Kinematics quaternions/DCM to quaternion/Case 3 ==
  A11 : Inport
  A22 : Inport  Port=2
  A33 : Inport  Port=3
  Add : Sum  Inputs=+--+
  Constant : Constant
  Gain : Gain  Gain=1/2
  Sqrt : Sqrt
  q3 : Outport
  wires:
  Gain/1 -> q3/1
  Sqrt/1 -> Gain/1
  Add/1 -> Sqrt/1
  Constant/1 -> Add/1
  A33/1 -> Add/4
  A11/1 -> Add/2
  A22/1 -> Add/3

== system main_model/Kinematics quaternions/DCM to quaternion/Case 4 ==
  A11 : Inport
  A22 : Inport  Port=2
  A33 : Inport  Port=3
  Add : Sum  Inputs=++++
  Constant : Constant
  Gain : Gain  Gain=1/2
  Sqrt : Sqrt
  q4 : Outport
  wires:
  A22/1 -> Add/3
  A11/1 -> Add/2
  A33/1 -> Add/4
  Constant/1 -> Add/1
  Add/1 -> Sqrt/1
  Sqrt/1 -> Gain/1
  Gain/1 -> q4/1

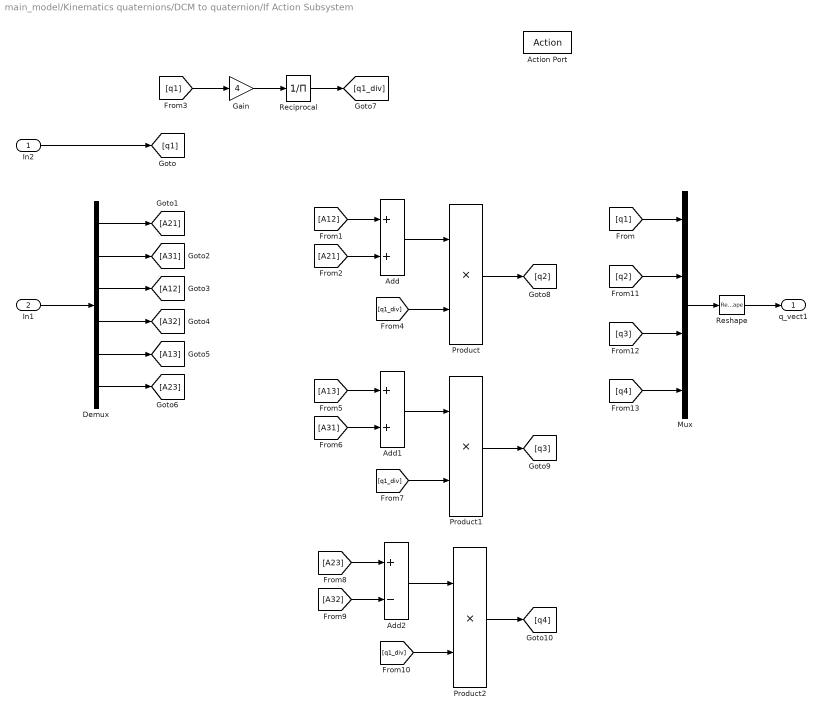
== system main_model/Kinematics quaternions/DCM to quaternion/If Action Subsystem ==
  In2 : Inport
  In1 : Inport  Port=2
  Action Port : ActionPort
  Add : Sum
  Add1 : Sum
  Add2 : Sum  Inputs=+-
  Demux : Demux  Outputs=6
  Gain : Gain  Gain=4
  Mux : Mux
  Product : Product
  Product1 : Product
  Product2 : Product
  Reciprocal : Product  Inputs=/
  Reshape : Reshape  OutputDimensionality=Column vector (2-D)
  q_vect1 : Outport
  wires:
  [q4] -> Mux/4
  [q3] -> Mux/3
  [q2] -> Mux/2
  Product2/1 -> [q4]
  [q1_div] -> Product2/2
  [A23] -> Add2/1
  [A32] -> Add2/2
  Add2/1 -> Product2/1
  Add1/1 -> Product1/1
  [A31] -> Add1/2
  [A13] -> Add1/1
  [q1_div] -> Product1/2
  Product1/1 -> [q3]
  Product/1 -> [q2]
  [q1_div] -> Product/2
  [A12] -> Add/1
  [A21] -> Add/2
  Add/1 -> Product/1
  Reciprocal/1 -> [q1_div]
  Gain/1 -> Reciprocal/1
  [q1] -> Gain/1
  Demux/4 -> [A32]
  Demux/5 -> [A13]
  Demux/6 -> [A23]
  Demux/1 -> [A21]
  Demux/2 -> [A31]
  Demux/3 -> [A12]
  [q1] -> Mux/1
  Reshape/1 -> q_vect1/1
  Mux/1 -> Reshape/1
  In2/1 -> [q1]
  In1/1 -> Demux/1

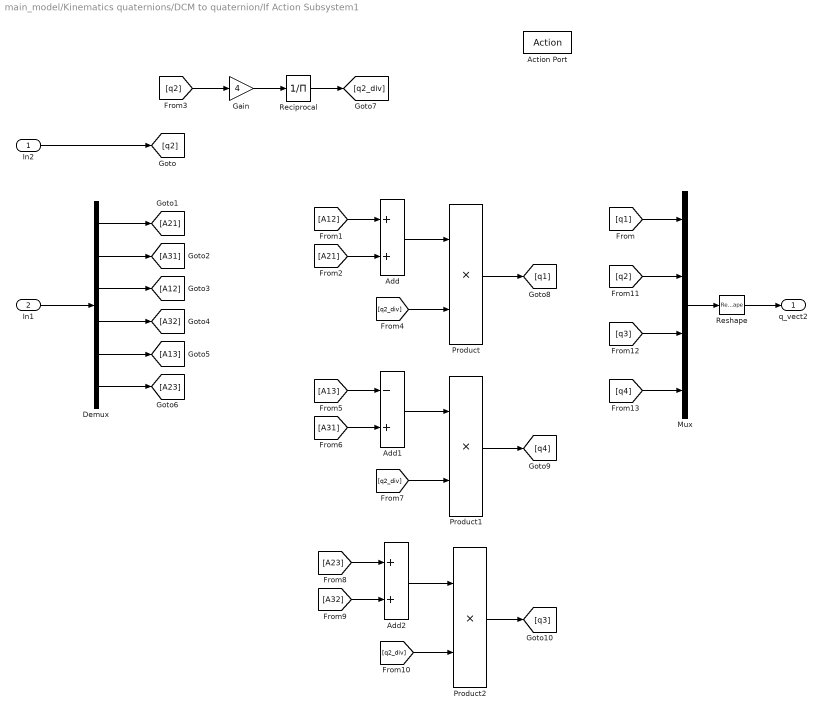
== system main_model/Kinematics quaternions/DCM to quaternion/If Action Subsystem1 ==
  In2 : Inport
  In1 : Inport  Port=2
  Action Port : ActionPort
  Add : Sum
  Add1 : Sum  Inputs=-+
  Add2 : Sum
  Demux : Demux  Outputs=6
  Gain : Gain  Gain=4
  Mux : Mux
  Product : Product
  Product1 : Product
  Product2 : Product
  Reciprocal : Product  Inputs=/
  Reshape : Reshape  OutputDimensionality=Column vector (2-D)
  q_vect2 : Outport
  wires:
  In1/1 -> Demux/1
  In2/1 -> [q2]
  Mux/1 -> Reshape/1
  Reshape/1 -> q_vect2/1
  [q1] -> Mux/1
  Demux/3 -> [A12]
  Demux/2 -> [A31]
  Demux/1 -> [A21]
  Demux/6 -> [A23]
  Demux/5 -> [A13]
  Demux/4 -> [A32]
  [q2] -> Gain/1
  Gain/1 -> Reciprocal/1
  Reciprocal/1 -> [q2_div]
  Add/1 -> Product/1
  [A21] -> Add/2
  [A12] -> Add/1
  [q2_div] -> Product/2
  Product/1 -> [q1]
  Product1/1 -> [q4]
  [q2_div] -> Product1/2
  [A13] -> Add1/1
  [A31] -> Add1/2
  Add1/1 -> Product1/1
  Add2/1 -> Product2/1
  [A32] -> Add2/2
  [A23] -> Add2/1
  [q2_div] -> Product2/2
  Product2/1 -> [q3]
  [q2] -> Mux/2
  [q3] -> Mux/3
  [q4] -> Mux/4

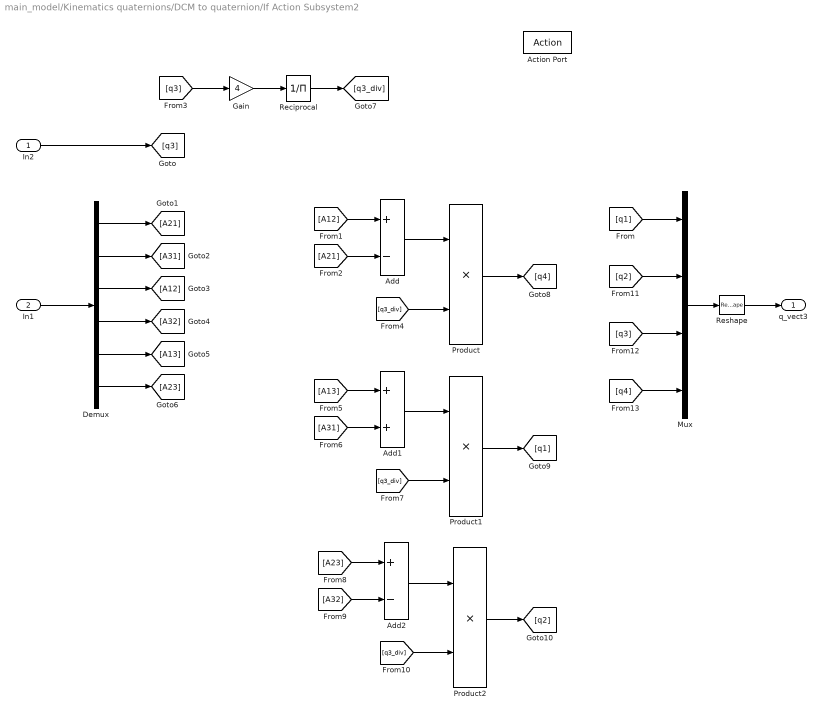
== system main_model/Kinematics quaternions/DCM to quaternion/If Action Subsystem2 ==
  In2 : Inport
  In1 : Inport  Port=2
  Action Port : ActionPort
  Add : Sum  Inputs=+-
  Add1 : Sum
  Add2 : Sum  Inputs=+-
  Demux : Demux  Outputs=6
  Gain : Gain  Gain=4
  Mux : Mux
  Product : Product
  Product1 : Product
  Product2 : Product
  Reciprocal : Product  Inputs=/
  Reshape : Reshape  OutputDimensionality=Column vector (2-D)
  q_vect3 : Outport
  wires:
  [q4] -> Mux/4
  [q3] -> Mux/3
  [q2] -> Mux/2
  Product2/1 -> [q2]
  [q3_div] -> Product2/2
  [A23] -> Add2/1
  [A32] -> Add2/2
  Add2/1 -> Product2/1
  Add1/1 -> Product1/1
  [A31] -> Add1/2
  [A13] -> Add1/1
  [q3_div] -> Product1/2
  Product1/1 -> [q1]
  Product/1 -> [q4]
  [q3_div] -> Product/2
  [A12] -> Add/1
  [A21] -> Add/2
  Add/1 -> Product/1
  Reciprocal/1 -> [q3_div]
  Gain/1 -> Reciprocal/1
  [q3] -> Gain/1
  Demux/4 -> [A32]
  Demux/5 -> [A13]
  Demux/6 -> [A23]
  Demux/1 -> [A21]
  Demux/2 -> [A31]
  Demux/3 -> [A12]
  [q1] -> Mux/1
  Reshape/1 -> q_vect3/1
  Mux/1 -> Reshape/1
  In2/1 -> [q3]
  In1/1 -> Demux/1

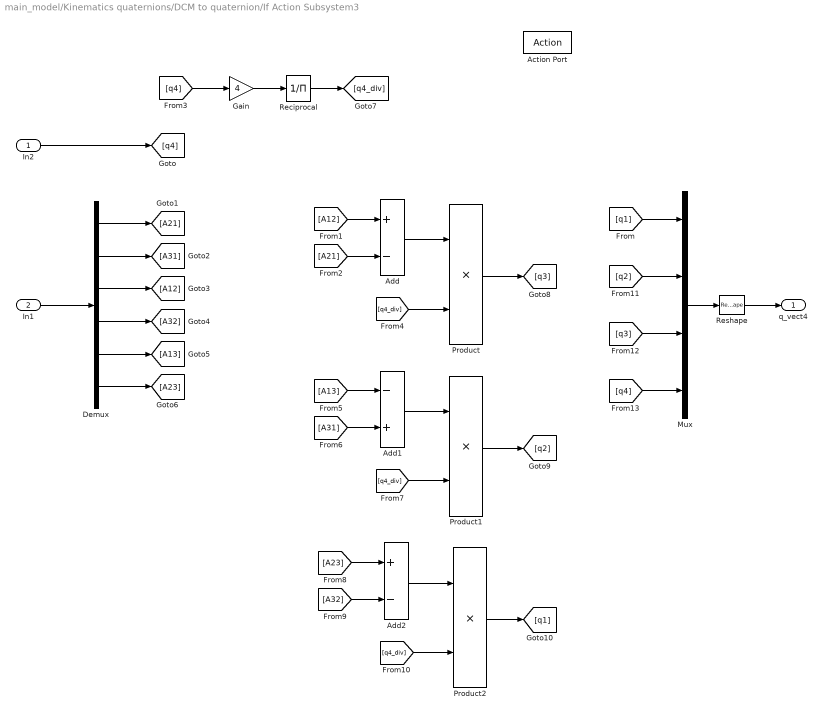
== system main_model/Kinematics quaternions/DCM to quaternion/If Action Subsystem3 ==
  In2 : Inport
  In1 : Inport  Port=2
  Action Port : ActionPort
  Add : Sum  Inputs=+-
  Add1 : Sum  Inputs=-+
  Add2 : Sum  Inputs=+-
  Demux : Demux  Outputs=6
  Gain : Gain  Gain=4
  Mux : Mux
  Product : Product
  Product1 : Product
  Product2 : Product
  Reciprocal : Product  Inputs=/
  Reshape : Reshape  OutputDimensionality=Column vector (2-D)
  q_vect4 : Outport
  wires:
  In1/1 -> Demux/1
  In2/1 -> [q4]
  Mux/1 -> Reshape/1
  Reshape/1 -> q_vect4/1
  [q1] -> Mux/1
  Demux/3 -> [A12]
  Demux/2 -> [A31]
  Demux/1 -> [A21]
  Demux/6 -> [A23]
  Demux/5 -> [A13]
  Demux/4 -> [A32]
  [q4] -> Gain/1
  Gain/1 -> Reciprocal/1
  Reciprocal/1 -> [q4_div]
  Add/1 -> Product/1
  [A21] -> Add/2
  [A12] -> Add/1
  [q4_div] -> Product/2
  Product/1 -> [q3]
  Product1/1 -> [q2]
  [q4_div] -> Product1/2
  [A13] -> Add1/1
  [A31] -> Add1/2
  Add1/1 -> Product1/1
  Add2/1 -> Product2/1
  [A32] -> Add2/2
  [A23] -> Add2/1
  [q4_div] -> Product2/2
  Product2/1 -> [q1]
  [q2] -> Mux/2
  [q3] -> Mux/3
  [q4] -> Mux/4

== system main_model/Kinematics quaternions/q to DCM/q cross ==
  q_vec : Inport
  Demux : Demux  Outputs=3
  Gain : Gain  Gain=-1
  Gain1 : Gain  Gain=-1
  Gain2 : Gain  Gain=-1
  Ground : Ground
  Reshape : Reshape  OutputDimensionality=Customize  OutputDimensions=[3,3]
  Vector Concatenate : Concatenate  NumInputs=9
  q cross : Outport
  wires:
  Gain2/1 -> Vector Concatenate/8
  [q1] -> Gain2/1
  [q2] -> Vector Concatenate/7
  [q1] -> Vector Concatenate/6
  [q3] -> Gain1/1
  Gain1/1 -> Vector Concatenate/4
  [q2] -> Gain/1
  Gain/1 -> Vector Concatenate/3
  [q3] -> Vector Concatenate/2
  Demux/3 -> [q3]
  Demux/2 -> [q2]
  Demux/1 -> [q1]
  q_vec/1 -> Demux/1
  Ground/1 -> Vector Concatenate/1, Vector Concatenate/5, Vector Concatenate/9
  Vector Concatenate/1 -> Reshape/1
  Reshape/1 -> q cross/1

== system main_model/External Torques/Solar radiation/Force MB/Subsystem ==
  S_B : Inport
  N_MB : Inport  Port=2
  Constant3 : Constant  Value=[1, 1, 1]
  Matrix Multiply5 : Product  Multiplication=Matrix(*)
  Product10 : Product
  Reshape11 : Reshape  OutputDimensionality=Row vector (2-D)
  Reshape12 : Reshape  OutputDimensionality=Column vector (2-D)
  Sum of Elements : Sum  Inputs=+  CollapseMode=Specified dimension  CollapseDim=2
  Out1 : Outport
  wires:
  Matrix Multiply5/1 -> Product10/1
  Reshape12/1 -> Matrix Multiply5/1
  S_B/1 -> Reshape12/1
  Product10/1 -> Sum of Elements/1
  N_MB/1 -> Product10/2
  Sum of Elements/1 -> Out1/1
  Constant3/1 -> Reshape11/1
  Reshape11/1 -> Matrix Multiply5/2

== system main_model/External Torques/Solar radiation/Inertia matrix/r_SP ==
  b_SP : Inport
  a_MB : Inport  Port=2
  Constant : Constant  Value=[1 0 0]
  Gain : Gain  Gain=1/2
  Gain1 : Gain  Gain=1/2
  Gain2 : Gain  Gain=-1
  Product : Product
  Reshape : Reshape  OutputDimensionality=Column vector (2-D)
  Sum : Sum
  r_SP1 : Outport
  r_SP2 : Outport  Port=2
  wires:
  Constant/1 -> Reshape/1
  a_MB/1 -> Gain/1
  b_SP/1 -> Gain1/1
  Gain1/1 -> Sum/1
  Gain/1 -> Sum/2
  Reshape/1 -> Product/1
  Sum/1 -> Product/2
  Gain2/1 -> r_SP2/1
  Product/1 -> r_SP1/1, Gain2/1
